simulink model "AMR_UDP_Joystick_24a"  (R2024a)
settings: configuration reference "SharedConfig" (kept outside this file)
undefined symbols (not defined in the file): tstep
libraries: slrealtimeutilitieslib x1
settings Model: DataDictionary=configuration_dictionary.sldd  Creator=matlab.cut  LastModifiedBy=ander
settings ConfigSetRef: SourceName=SharedConfig

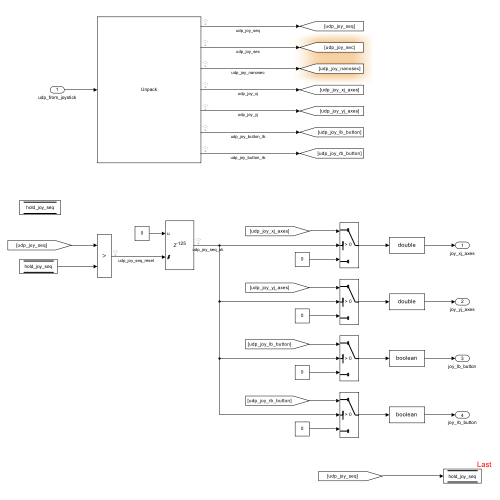
[thumbnail: Simulink's stored preview of the top-level diagram]
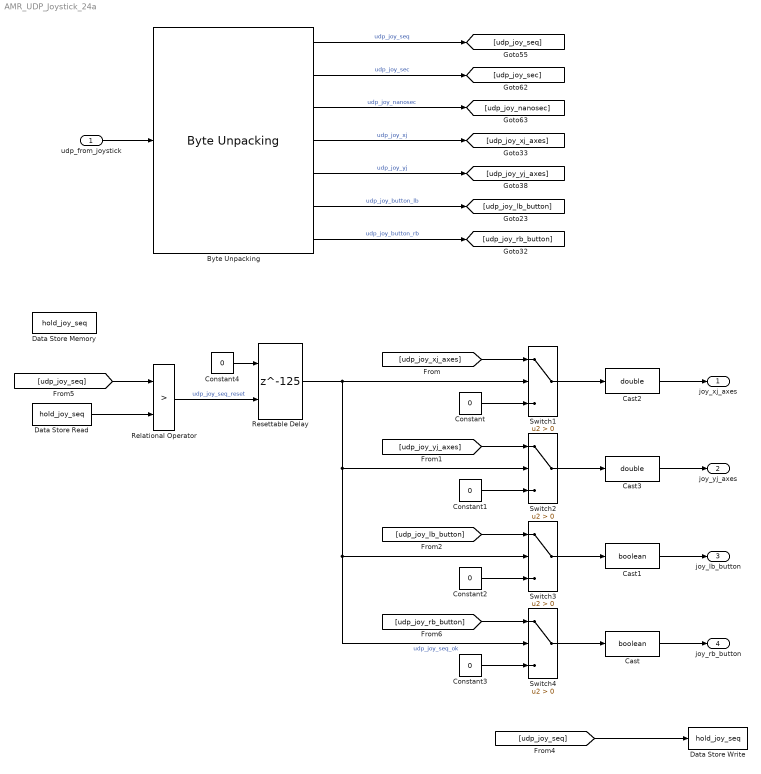
== system AMR_UDP_Joystick_24a ==
  udp_from_joystick : Inport  OutDataTypeStr=uint8  PortDimensions=36
  Byte Unpacking : slrealtimeutilitieslib/Byte Unpacking  MaskUnpackedDataTypes={'uint32','double','double','single','single','int32','int32'}  MaskUnpackedDataSizes={[1],[1],[1],[1],[1],[1],[1]}  MaskAlignment=1
  Cast : DataTypeConversion  OutDataTypeStr=boolean  SaturateOnIntegerOverflow=off  RndMeth=Floor
  Cast1 : DataTypeConversion  OutDataTypeStr=boolean  SaturateOnIntegerOverflow=off  RndMeth=Floor
  Cast2 : DataTypeConversion  OutDataTypeStr=double  SaturateOnIntegerOverflow=off  RndMeth=Floor
  Cast3 : DataTypeConversion  OutDataTypeStr=double  SaturateOnIntegerOverflow=off  RndMeth=Floor
  Constant{,1..4} (5 alike) : Constant  Value=0
  Data Store Memory : DataStoreMemory  DataStoreName=hold_joy_seq  WriteAfterWriteMsg=warning  ShowAdditionalParam=off  OutDataTypeStr=uint32  Dimensions=1
      settings: LockScale=on
  Data Store Read : DataStoreRead  DataStoreName=hold_joy_seq  DataStoreElements=hold_joy_seq  IndexOptions=Index vector (dialog)  Indices=1  OutputSizes=1
  Data Store Write : DataStoreWrite  ExecutionOrder=Last  DataStoreName=hold_joy_seq  DataStoreElements=hold_joy_seq  IndexOptions=Index vector (dialog)  Indices=1  OutputSizes=1
  Relational Operator : RelationalOperator  Operator=>  OutDataTypeStr=boolean  RndMeth=Simplest  InputSameDT=off
  Resettable Delay : Delay  DelayLength=125  InitialCondition=1  ExternalReset=Rising  SampleTime=tstep
      settings: InputPortMap=u0,r5
  Switch{1..4} (4 alike) : Switch  Criteria=u2 > Threshold  SaturateOnIntegerOverflow=off  InputSameDT=off
  joy_xj_axes : Outport  OutDataTypeStr=double
  joy_yj_axes : Outport  Port=2  OutDataTypeStr=double
  joy_lb_button : Outport  Port=3  OutDataTypeStr=boolean
  joy_rb_button : Outport  Port=4  OutDataTypeStr=boolean
  wires:
  Byte Unpacking/3 -> [udp_joy_nanosec]  "udp_joy_nanosec"
  udp_from_joystick/1 -> Byte Unpacking/1
  Byte Unpacking/4 -> [udp_joy_xj_axes]  "udp_joy_xj"
  Byte Unpacking/6 -> [udp_joy_lb_button]  "udp_joy_button_lb"
  Byte Unpacking/1 -> [udp_joy_seq]  "udp_joy_seq"
  Byte Unpacking/7 -> [udp_joy_rb_button]  "udp_joy_button_rb"
  Byte Unpacking/2 -> [udp_joy_sec]  "udp_joy_sec"
  Byte Unpacking/5 -> [udp_joy_yj_axes]  "udp_joy_yj"
  Switch4/1 -> Cast/1
  Cast/1 -> joy_rb_button/1
  Cast1/1 -> joy_lb_button/1
  Cast2/1 -> joy_xj_axes/1
  Cast3/1 -> joy_yj_axes/1
  [udp_joy_seq] -> Data Store Write/1
  [udp_joy_seq] -> Relational Operator/1
  Data Store Read/1 -> Relational Operator/2
  [udp_joy_xj_axes] -> Switch1/1
  Switch1/1 -> Cast2/1
  Constant/1 -> Switch1/3
  Constant1/1 -> Switch2/3
  [udp_joy_yj_axes] -> Switch2/1
  Switch2/1 -> Cast3/1
  Constant2/1 -> Switch3/3
  [udp_joy_lb_button] -> Switch3/1
  Switch3/1 -> Cast1/1
  [udp_joy_rb_button] -> Switch4/1
  Constant3/1 -> Switch4/3
  Relational Operator/1 -> Resettable Delay/2  "udp_joy_seq_reset"
  Constant4/1 -> Resettable Delay/1
  Resettable Delay/1 -> Switch4/2, Switch3/2, Switch2/2, Switch1/2  "udp_joy_seq_ok"
